simulink model "aero_bf_simu"  (R2019a)
settings: Solver=ode5  StartTime=0.0  StopTime=600  FixedStep=Ts  RelTol=1e-3
values from neighbouring files (symbols this model uses):
  k1 = 0.78    [Aero_init.m]    (also in aide_resolution_eq_bezout.m)
  k2 = -0.25    [Aero_init.m]    (also in aide_resolution_eq_bezout.m)
  R = [r0 r1 r2]    [Aero_init.m]    (also in aide_resolution_eq_bezout.m = [ r0 r1 r2])
  S = [1 s-1 -s]    [Aero_init.m]    (also in aide_resolution_eq_bezout.m = [ 1 sp1-1 -sp1])
  T = [r0+r1+r2]    [Aero_init.m]    (also in aide_resolution_eq_bezout.m = [ r0+r1+r2 ])
  tau = 7.64    [Aero_init.m]    (also in aide_resolution_eq_bezout.m)
  Te = 2.0    (= 2)    [Aero_init.m]    (also in aide_resolution_eq_bezout.m)
  Ts = 0.1    [Aero_init.m]    (also in aide_resolution_eq_bezout.m)
  U0 = 5    [Aero_init.m]    (also in aide_resolution_eq_bezout.m)
settings Model: ExtModeTrigDuration=6000  Creator=drey  LastModifiedBy=DELL
settings DataIOCC: SaveFormat=Array  SignalLoggingSaveFormat=ModelDataLogs  ReturnWorkspaceOutputs=off
settings OptimizationCC: BlockReduction=off  BooleanDataType=off  ExpressionDepthLimit=2147483647  InitFltsAndDblsToZero=on  LifeSpan=1
settings DebuggingCC: SaveWithParameterizedLinksMsg=none  UnderspecifiedInitializationDetection=Classic  MergeDetectMultiDrivingBlocksExec=none  SignalResolutionControl=TryResolveAllWithWarning  MultiTaskDSMMsg=warning  MultiTaskCondExecSysMsg=none  FcnCallInpInsideContextMsg=warning  StateNameClashWarn=warning  SFUnexpectedBacktrackingDiag=warning  SFNoUnconditionalDefaultTransitionDiag=warning  SFExecutionAtInitializationDiag=none  ArithmeticOperatorsInVariantConditions=warning
settings HardwareCC: ProdBitPerPointer=32  ProdBitPerSizeT=32  ProdBitPerPtrDiffT=32  ProdLargestAtomicFloat=None  ProdIntDivRoundTo=Undefined  ProdEndianess=Unspecified  ProdWordSize=32  ProdHWDeviceType=32-bit Generic
settings ModelReferenceCC: PropagateSignalLabelsOutOfModel=off
settings SFSimCC: SimUseLocalCustomCode=off  MATLABDynamicMemAlloc=off
settings RTWCC: SystemTargetFile=ert.tlc  TemplateMakefile=ert_msvc.tmf  Description=Visual C/C++ Project Makefile only for the Real-Time Workshop Embedded Coder  RTWUseLocalCustomCode=off
settings CodeAppCC: IgnoreCustomStorageClasses=off  CustomSymbolStrType=$N$R$M  StateflowObjectComments=on  InternalIdentifier=Classic
settings ERTTargetCC: GenerateSampleERTMain=on  ERTCustomFileTemplate=example_file_process.tlc  ConvertIfToSwitch=off  SuppressUnreachableDefaultCases=off
settings ConfigComp: CovMetricSettings=dw  CovHtmlReporting=on  CovSaveCumulativeToWorkspaceVar=on  CovSaveSingleToWorkspaceVar=on  CovExternalEMLEnable=off

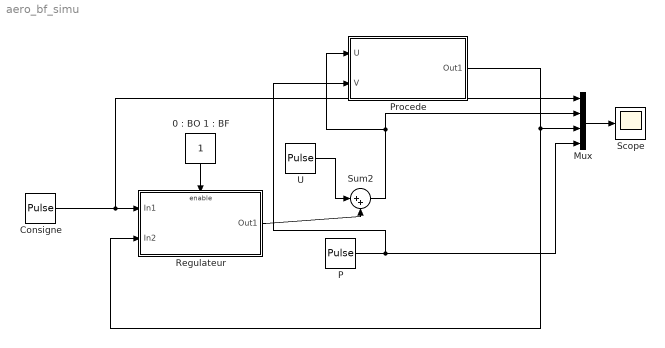
== system aero_bf_simu ==
  "0 : BO 1 : BF" : Constant
  Consigne : DiscretePulseGenerator  PulseType=Time based  Period=200  PulseWidth=50  PhaseDelay=100
  Mux : Mux
  P : DiscretePulseGenerator  PulseType=Time based  Amplitude=0  Period=200  PulseWidth=50  PhaseDelay=150
  Procede : Subsystem
      mask Display: disp('Procede')
  Regulateur : Subsystem  TreatAsAtomicUnit=on
      mask Display: disp('Regulateur')
  Scope : Scope
  Sum2 : Sum  Inputs=|++  SaturateOnIntegerOverflow=on  InputSameDT=on  OutDataTypeStr=Inherit: Same as first input
  U : DiscretePulseGenerator  PulseType=Time based  Amplitude=0  Period=200  PulseWidth=50  PhaseDelay=100
  wires:
  Consigne/1 -> Mux/1, Regulateur/1(In1)
  "0 : BO 1 : BF"/1 -> Regulateur/Enable
  U/1 -> Sum2/1
  Regulateur/1(Out1) -> Sum2/2
  Sum2/1 -> Mux/2, Procede/1(U)
  Mux/1 -> Scope/1
  Procede/1(Out1) -> Regulateur/2(In2), Mux/3
  P/1 -> Mux/4, Procede/2(V)

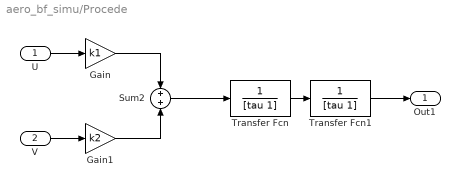
== system aero_bf_simu/Procede ==
  U : Inport
  V : Inport  Port=2
  Gain : Gain  Gain=k1
  Gain1 : Gain  Gain=k2
  Sum2 : Sum  Inputs=+|+  SaturateOnIntegerOverflow=on  InputSameDT=on  OutDataTypeStr=Inherit: Same as first input
  Transfer Fcn : TransferFcn  Denominator=[tau 1]
  Transfer Fcn1 : TransferFcn  Denominator=[tau 1]
  Out1 : Outport
  wires:
  Transfer Fcn1/1 -> Out1/1
  Transfer Fcn/1 -> Transfer Fcn1/1
  Sum2/1 -> Transfer Fcn/1
  U/1 -> Gain/1
  Gain/1 -> Sum2/1
  V/1 -> Gain1/1
  Gain1/1 -> Sum2/2

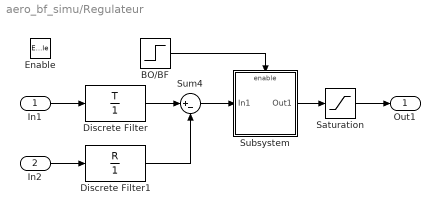
== system aero_bf_simu/Regulateur ==
  In1 : Inport
  In2 : Inport  Port=2
  Enable : EnablePort
  BO/BF : Step  Time=10  SampleTime=Ts
  Discrete Filter : DiscreteFilter  Numerator=T  Denominator=1  SampleTime=Te
  Discrete Filter1 : DiscreteFilter  Numerator=R  Denominator=1  SampleTime=Te
  Saturation : Saturate  UpperLimit=10-U0  LowerLimit=0-U0
  Subsystem : Subsystem  TreatAsAtomicUnit=on
      mask Display: disp('1/S(z)')
  Sum4 : Sum  Inputs=|+-  SaturateOnIntegerOverflow=on  InputSameDT=on  OutDataTypeStr=Inherit: Same as first input
  Out1 : Outport
  wires:
  BO/BF/1 -> Subsystem/Enable
  Discrete Filter1/1 -> Sum4/2
  In2/1 -> Discrete Filter1/1
  Saturation/1 -> Out1/1
  Subsystem/1(Out1) -> Saturation/1
  In1/1 -> Discrete Filter/1
  Discrete Filter/1 -> Sum4/1
  Sum4/1 -> Subsystem/1(In1)

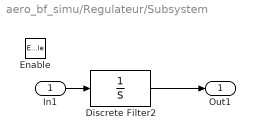
== system aero_bf_simu/Regulateur/Subsystem ==
  In1 : Inport
  Enable : EnablePort
  Discrete Filter2 : DiscreteFilter  Numerator=1  Denominator=S  SampleTime=Te
  Out1 : Outport
  wires:
  Discrete Filter2/1 -> Out1/1
  In1/1 -> Discrete Filter2/1
